simulink model "bike_model_old"  (R2018b)
settings: Solver=VariableStepAuto  StartTime=0.0  StopTime=sim_time  FixedStep=Ts_IMU  MaxStep=Ts  RelTol=1e-3
values from neighbouring files (symbols this model uses):
  a_compFilter = b_compFilter - 0.77    (= 0.325)    [configuration.m]    (also in configuration_pidTuning.m)
  A_kalman = [1 0 Ts 0; 0 1 0 Ts; 0 0 1 0; 0 0 0 1]    [configuration.m]    (also in configuration_pidTuning.m)
  b_compFilter = 1.095    [configuration.m]    (also in configuration_pidTuning.m)
  B_kalman = [0 0 0 0; 0 0 0 0; 0 0 0 0; 0 0 0 0]    [configuration.m]    (also in configuration_pidTuning.m)
  b_real = 1.095    [configuration.m]    (also in configuration_pidTuning.m)
  C_kalman = [1 0 0 0; 0 1 0 0; 0 0 1 0; 0 0 0 1]    [configuration.m]    (also in configuration_pidTuning.m)
  complementary = 0.985    [configuration.m]    (also in configuration_pidTuning.m)
  D_kalman = [0 0 0 0; 0 0 0 0; 0 0 0 0; 0 0 0 0]    [configuration.m]    (also in configuration_pidTuning.m)
  Dead_Band = [0.055, -0.055, 0.005]    [configuration.m]    (also in configuration_pidTuning.m)
  delay = 0.045    [configuration.m]    (also in configuration_pidTuning.m)
  direct_control = 1    [configuration.m]    (also in configuration_pidTuning.m)
  filter_model = 1    [configuration.m]    (also in configuration_pidTuning.m)
  forward_motor_dynamics = 0    [configuration.m]    (also in configuration_pidTuning.m)
  forward_speed_offset = 0    [configuration.m]
  g = 9.81    [configuration.m]    (also in configuration_pidTuning.m)
  I_direct = 0.000227125326188444    (= 0.000227125326188)    [configuration.m]    (also in configuration_pidTuning.m)
  I_lat = 0.000115580509653549    (= 0.000115580509654)    [configuration.m]    (also in configuration_pidTuning.m)
  I_steer = 0.4510120195392    (= 0.451012019539)    [configuration.m]    (also in configuration_pidTuning.m)
  IMU_height_model = 0.45    [configuration.m]    (also in configuration_pidTuning.m)
  IMU_height_real = 0.45    [configuration.m]    (also in configuration_pidTuning.m)
  initial_states = [deg2rad(-2) deg2rad(0) deg2rad(0)]    [configuration.m]    (also in configuration_pidTuning.m)
  input_velocity = 4    [configuration.m]    (also in configuration_pidTuning.m = 3)
  K_dir = [0.2 0 0]    [configuration.m]
  K_pos = [0.02 0 0]    [configuration.m]
  lambda_compFilter = deg2rad(70)    [configuration.m]    (also in configuration_pidTuning.m)
  lambda_real = deg2rad(70)    [configuration.m]    (also in configuration_pidTuning.m)
  lat_control = 0    [configuration.m]    (also in configuration_pidTuning.m = 1)
  look_ahead = 0    [configuration.m]    (also in configuration_pidTuning.m)
  lqr_gains = zeros(length(velocity_lqr),1+size(A_bike,1))    [lqr_design.m]
  max_handlebar = 40*(pi/180)    (= 0.698131700798)    [configuration.m]    (also in configuration_pidTuning.m)
  max_roll = pi/2    (= 1.57079632679)    [configuration.m]    (also in configuration_pidTuning.m)
  max_steering_motor_acc = inf    [configuration.m]    (also in configuration_pidTuning.m)
  max_steering_motor_speed = 0.9    [configuration.m]    (also in configuration_pidTuning.m = 7.5)
  min_handlebar = -max_handlebar    (= -0.698131700798)    [configuration.m]    (also in configuration_pidTuning.m)
  min_roll = - max_roll    (= -1.57079632679)    [configuration.m]    (also in configuration_pidTuning.m)
  min_steering_motor_acc = -inf    [configuration.m]    (also in configuration_pidTuning.m)
  min_steering_motor_speed = -0.9    [configuration.m]    (also in configuration_pidTuning.m = -7.5)
  noise = 0    [configuration.m]    (also in configuration_pidTuning.m)
  noise_acc = 2.4869e-05    [configuration.m]    (also in configuration_pidTuning.m)
  noise_encoder = 1e-7    (= 1e-07)    [configuration.m]    (also in configuration_pidTuning.m)
  noise_gyro = 0.005    [configuration.m]    (also in configuration_pidTuning.m = 0.0022)
  noise_hall = 0.0031    [configuration.m]    (also in configuration_pidTuning.m)
  noise_pos_meas = 0    [configuration.m]    (also in configuration_pidTuning.m = 0.51)
  offset_acc = 0.0*g    (= 0)    [configuration.m]
  offset_encoder = deg2rad(1)    [configuration.m]
  offset_gyro = deg2rad(0)    [configuration.m]
  offset_hall = 0.0    (= 0)    [configuration.m]
  offset_pos_x = 0    [configuration.m]
  offset_pos_y = 0    [configuration.m]
  P_direct = 0.0712859744206787    (= 0.0712859744207)    [configuration.m]    (also in configuration_pidTuning.m)
  P_lat = 0.0465435246389258    (= 0.0465435246389)    [configuration.m]    (also in configuration_pidTuning.m)
  P_steer = 0.219020351848633    (= 0.219020351849)    [configuration.m]    (also in configuration_pidTuning.m)
  parameters_compFilter = [g h_compFilter b_compFilter a_compFilter lambda_compFilter c_compFilter]    [configuration.m]    (also in configuration_pidTuning.m)
  parameters_f_b_real = [m_frame_real m_box_real h_frame_real h_box_real a_frame_real a_box_real c_frame_real c_box_real b_frame_real b_box_real l_frame_real l_box_real]    [configuration.m]    (also in configuration_pidTuning.m)
  parameters_real = [g h_real b_real a_real lambda_real c_real]    [configuration.m]    (also in configuration_pidTuning.m)
  path_tracking = 0    [configuration.m]    (also in configuration_pidTuning.m = 1)
  plant_model = 2    [configuration.m]    (also in configuration_pidTuning.m = 1)
  R_kalman = [noise_pos_meas 0 0 0; 0 noise_pos_meas 0 0; 0 0 noise_hall 0; 0 0 0 noise_hall]    [configuration.m]    (also in configuration_pidTuning.m)
  roll_rate_coef = 0.9    [configuration.m]    (also in configuration_pidTuning.m)
  sensor_offset = 0    [configuration.m]
  steer_control = 0    [configuration.m]    (also in configuration_pidTuning.m = 1)
  steering_angle_correction = deg2rad(0)    [configuration.m]
  steering_motor_limitations = 0    [configuration.m]    (also in configuration_pidTuning.m = 1)
  sys_con = ss(A_lqr,B_lqr,C_lqr,D_lqr)    [lqr_design.m]
  sys_dis = c2d(sys_con,Ts)    [lqr_design.m]
  time_offset_acc = 7    [configuration.m]
  time_offset_encoder = 10    [configuration.m]
  time_offset_gyro = 7    [configuration.m]
  time_offset_hall = 7    [configuration.m]
  time_offset_pos_x = 7    [configuration.m]
  time_offset_pos_y = 7    [configuration.m]
  Ts = 0.01    [configuration.m]    (also in configuration_pidTuning.m = 0.04)
  Ts_IMU = 0.01    [configuration.m]    (also in configuration_pidTuning.m = 0.04)
  uneven_mass = 0    [configuration.m]
  velocity_lqr = [input_velocity - 0.1 , input_velocity , input_velocity + 0.1]    [lqr_design.m]
undefined symbols (not defined in the file or in its folder): A, B, cumulative_dist_along_path, curvature, DiscIntNeverNeededParam, Discrete, initial_x, initial_y, path_x, path_y, Time
libraries: simulink x23, simulink_extras x4, dspsigops x2, ctrlSharedLib x1
(part 3 of 3)

== system bike_model_old/Reference Position /Variable Look Ahead ==
  Velocity : Inport
  Total Tavelled Distance : Inport  Port=2
  1-D Lookup Table2 : Lookup_n-D  NumberOfTableDimensions=1  BreakpointsForDimension1=cumulative_dist_along_path  Table=curvature  ExtrapMethod=Clip  DiagnosticForOutOfRangeInput=Error  InternalRulePriority=Speed  RndMeth=Simplest  InputSameDT=on
  Add1 : Sum
  Clock : Clock
  Delay : Delay  DelayLength=1
  Delay1 : Delay  DelayLength=1
  Demux3 : Demux  Outputs=2
  Gain : Gain  Gain=8
  Look Ahead Time for Curvature Check : Gain  Gain=3
  Look-Ahead Coefficient Selector : MATLAB Function  TreatAsAtomicUnit=on
  "Look-Ahead Coefficient Modifier (Slow Turn-Off) " : MATLAB Function  TreatAsAtomicUnit=on
  Mux1 : Mux  Inputs=2
  Product3 : Product
  Scope2 : Scope
  Look Ahead Distance : Outport
  wires:
  Look Ahead Time for Curvature Check/1 -> Add1/1
  Delay/1 -> "Look-Ahead Coefficient Modifier (Slow Turn-Off) "/2(feedback)
  "Look-Ahead Coefficient Modifier (Slow Turn-Off) "/1(look_ahead_modified) -> Delay/1, Gain/1
  Demux3/1 -> Look-Ahead Coefficient Selector/1(curv_next)
  Look-Ahead Coefficient Selector/1(look_ahead) -> "Look-Ahead Coefficient Modifier (Slow Turn-Off) "/1(look_ahead), Scope2/1
  Clock/1 -> "Look-Ahead Coefficient Modifier (Slow Turn-Off) "/3(time), Delay1/1
  Delay1/1 -> "Look-Ahead Coefficient Modifier (Slow Turn-Off) "/4(time_delayed)
  1-D Lookup Table2/1 -> Demux3/1
  Total Tavelled Distance/1 -> Add1/2, Mux1/2
  Demux3/2 -> Look-Ahead Coefficient Selector/2(curv)
  Gain/1 -> Product3/1  "Look-Ahead Time"
  Add1/1 -> Mux1/1
  Mux1/1 -> 1-D Lookup Table2/1
  Velocity/1 -> Product3/2, Look Ahead Time for Curvature Check/1
  Product3/1 -> Look Ahead Distance/1

== system bike_model_old/Steering Motor/Motor Deadband ==
  Calculated Input : Inport
  Abs : Abs
  Abs1 : Abs
  Constant : Constant  Value=0  SampleTime=Ts
  Constant1 : Constant  Value=0  SampleTime=Ts
  Constant2 : Constant  Value=Dead_Band(2)  SampleTime=Ts
  Constant4 : Constant  Value=Dead_Band(1)  SampleTime=Ts
  Gain : Gain  Gain=-1
  Relay1 : Relay  OnSwitchValue=Dead_Band(3)  OffSwitchValue=-Dead_Band(3)
  Relay2 : Relay  OnSwitchValue=Dead_Band(3)  OffSwitchValue=-Dead_Band(3)
  Sum1 : Sum  Inputs=-+|
  Sum2 : Sum  Inputs=-+|
  Switch : Switch  Criteria=u2 > Threshold
  Switch1 : Switch  Criteria=u2 > Threshold
  Switch2 : Switch  Criteria=u2 > Threshold
  Input Signal After Dead Band : Outport
  wires:
  Constant4/1 -> Sum1/1
  Sum1/1 -> Relay1/1
  Relay1/1 -> Switch/2
  Switch/1 -> Switch1/1
  Constant/1 -> Switch/3
  Switch1/1 -> Input Signal After Dead Band/1
  Switch2/1 -> Switch1/3
  Constant1/1 -> Switch2/3
  Gain/1 -> Sum2/1
  Calculated Input/1 -> Abs/1, Switch2/1, Abs1/1, Switch/1, Switch1/2
  Sum2/1 -> Relay2/1
  Relay2/1 -> Switch2/2
  Abs/1 -> Sum2/2
  Abs1/1 -> Sum1/2
  Constant2/1 -> Gain/1

== system bike_model_old/Steering Motor/Velocity Saturation wrt Max and Min Handle Bar Angles ==
  Reference Steering Rate : Inport
  States : Inport  Port=2
  AND : Logic  IconShape=distinctive  AllPortsSameDT=off  OutDataTypeStr=boolean
  AND1 : Logic  IconShape=distinctive  AllPortsSameDT=off  OutDataTypeStr=boolean
  Compare To Constant : simulink/Logic and Bit Operations/Compare To Constant  relop=>=  const=max_handlebar  OutDataTypeStr=boolean
  Compare To Constant1 : simulink/Logic and Bit Operations/Compare To Constant  relop=<=  const=min_handlebar  OutDataTypeStr=boolean
  Compare To Zero : simulink/Logic and Bit Operations/Compare To Zero  relop=>=  OutDataTypeStr=boolean
  Compare To Zero1 : simulink/Logic and Bit Operations/Compare To Zero  relop=<=  OutDataTypeStr=boolean
  Constant : Constant  Value=0
  Demux : Demux  Outputs=3
  OR : Logic  Operator=OR  IconShape=distinctive  AllPortsSameDT=off  OutDataTypeStr=boolean
  Switch : Switch  Criteria=u2 > Threshold
  Output Steering Rate : Outport
  wires:
  Switch/1 -> Output Steering Rate/1
  Constant/1 -> Switch/1
  States/1 -> Demux/1
  Compare To Constant/1 -> AND/2
  OR/1 -> Switch/2
  Reference Steering Rate/1 -> Switch/3, Compare To Zero/1, Compare To Zero1/1
  Compare To Constant1/1 -> AND1/1
  AND1/1 -> OR/2
  Demux/2 -> Compare To Constant/1, Compare To Constant1/1
  AND/1 -> OR/1
  Compare To Zero1/1 -> AND1/2
  Compare To Zero/1 -> AND/1

== system bike_model_old/Complementary filter/Roll Angle Estimation of Accelerometer/Centripetal Acceleration Compensator ==
  Steering Angle : Inport
  Velocity : Inport  Port=2
  Bike Model b : Constant  Value=b_compFilter
  Divide : Product  Inputs=*/
  Gain : Gain  Gain=sin(lambda_compFilter)
  Multiply : Product
  Square : Math  Operator=square  SaturateOnIntegerOverflow=on
  Tan : Trigonometry  Operator=tan
  Estimated Centripetal Acceleration : Outport
  wires:
  Velocity/1 -> Square/1
  Square/1 -> Divide/1
  Bike Model b/1 -> Divide/2
  Steering Angle/1 -> Gain/1
  Divide/1 -> Multiply/1
  Tan/1 -> Multiply/2
  Multiply/1 -> Estimated Centripetal Acceleration/1
  Gain/1 -> Tan/1

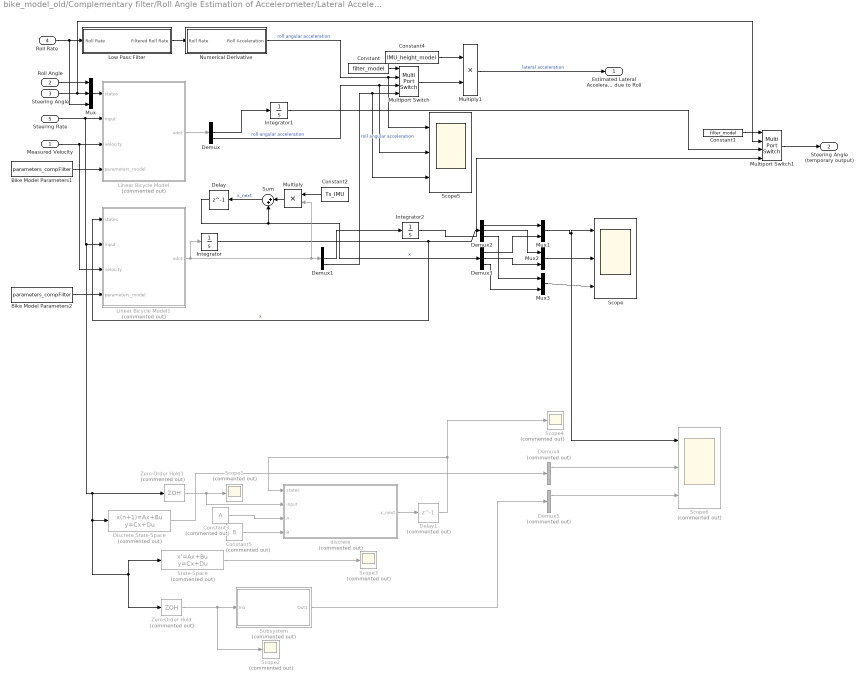
== system bike_model_old/Complementary filter/Roll Angle Estimation of Accelerometer/Lateral Acceleration Compensator ==
  Measured Velocity : Inport
  Roll Angle : Inport  Port=2
  Steering Angle : Inport  Port=3
  Roll Rate : Inport  Port=4
  Steering Rate : Inport  Port=5
  Bike Model Parameters1 : Constant  Value=parameters_compFilter
  Bike Model Parameters2 : Constant  Value=parameters_compFilter
  Constant : Constant  Value=filter_model
  Constant1 : Constant  Value=filter_model
  Constant2 : Constant  Value=Ts_IMU  SampleTime=Ts_IMU
  Constant3 : Constant  Commented=on  Value=A
  Constant4 : Constant  Value=IMU_height_model
  Constant5 : Constant  Commented=on  Value=B
  Delay : Delay  DelayLength=1  InitialCondition=[0 0 0]  SampleTime=Ts_IMU
  Delay1 : Delay  Commented=on  DelayLength=1  InitialCondition=[0 0 0]  SampleTime=Ts_IMU
  Demux{,1..3} (4 alike) : Demux  Outputs=3
  Demux4 : Demux  Commented=on  Outputs=3
  Demux5 : Demux  Commented=on  Outputs=3
  Discrete State-Space : DiscreteStateSpace  Commented=on  A=A  B=B  C=eye(3,3)  D=zeros(3,1)  InitialCondition=[0 0 0]  SampleTime=Ts_IMU
  Integrator : Integrator  InitialCondition=initial_states
  Integrator1 : Integrator  InitialCondition=initial_states(2)
  Integrator2 : Integrator  InitialCondition=initial_states(2)
  Linear Bicycle Model : MATLAB Function  Commented=on  TreatAsAtomicUnit=on
  Linear Bicycle Model1 : MATLAB Function  Commented=on  TreatAsAtomicUnit=on
  Low Pass Filter : Subsystem
  Multiply : Product
  Multiply1 : Product
  Multiport Switch : MultiPortSwitch
  Multiport Switch1 : MultiPortSwitch
  Mux : Mux  Inputs=3
  Mux1 : Mux  Inputs=2
  Mux2 : Mux  Inputs=2
  Mux3 : Mux  Inputs=2
  Numerical Derivative : Subsystem
  Scope : Scope  NumInputPorts=3
  Scope{1..4} (4 alike) : Scope  Commented=on
  Scope5 : Scope  NumInputPorts=3
  Scope6 : Scope  Commented=on  NumInputPorts=3
  State-Space : StateSpace  Commented=on  A=sys_con.A  B=sys_con.B  C=eye(3,3)  D=zeros(3,1)  InitialCondition=[0 0 0]
  Subsystem : Subsystem  Commented=on  TreatAsAtomicUnit=on  SystemSampleTime=Ts_IMU
  Sum : Sum  Inputs=|++
  Zero-Order Hold : ZeroOrderHold  Commented=on  SampleTime=Ts_IMU
  Zero-Order Hold1 : ZeroOrderHold  Commented=on  SampleTime=Ts_IMU
  discrete : MATLAB Function  Commented=on  TreatAsAtomicUnit=on
  Estimated Lateral Accelerattion due to Roll : Outport
  Steering Angle (temporary output) : Outport  Port=2
  wires:
  Numerical Derivative/1(Roll Acceleration) -> Scope5/1, Multiport Switch/2  "roll angular acceleration"
  Roll Rate/1 -> Mux/3, Low Pass Filter/1(Roll Rate)
  Constant4/1 -> Multiply1/1
  Multiply1/1 -> Estimated Lateral Accelerattion due to Roll/1  "lateral acceleration"
  Low Pass Filter/1(Filtered Roll Rate) -> Numerical Derivative/1(Roll Rate)
  Linear Bicycle Model/1(xdot) -> Demux/1
  Demux/3 -> Scope5/2, Multiport Switch/3  "roll angular acceleration"
  Bike Model Parameters1/1 -> Linear Bicycle Model/4(parameters_model)
  Measured Velocity/1 -> Linear Bicycle Model1/3(velocity), Linear Bicycle Model/3(velocity)
  Mux/1 -> Linear Bicycle Model/1(states)
  Roll Angle/1 -> Mux/1
  Steering Angle/1 -> Multiport Switch1/2, Mux/2
  Constant/1 -> Multiport Switch/1
  Multiport Switch/1 -> Multiply1/2
  Demux1/3 -> Scope5/3, Multiport Switch/4  "roll angular acceleration"
  Bike Model Parameters2/1 -> Linear Bicycle Model1/4(parameters_model)
  Delay/1 -> Demux3/1, Sum/2  "x"
  Multiply/1 -> Sum/1
  Constant2/1 -> Multiply/1
  Integrator/1 -> Linear Bicycle Model1/1(states), Demux2/1  "x"
  Demux2/1 -> Mux1/1
  Demux3/1 -> Mux1/2
  Demux2/2 -> Mux2/1
  Demux3/2 -> Mux2/2
  Demux2/3 -> Mux3/1
  Demux3/3 -> Mux3/2
  Mux2/1 -> Scope/2
  Mux1/1 -> Scope6/1, Scope/1
  Mux3/1 -> Scope/3
  Linear Bicycle Model1/1(xdot) -> Multiply/2, Demux1/1, Integrator/1
  State-Space/1 -> Scope3/1
  Delay1/1 -> Scope4/1, discrete/1(states)
  Zero-Order Hold/1 -> Scope2/1, Subsystem/1(In1)
  discrete/1(x_next) -> Delay1/1
  Constant5/1 -> discrete/4(B)
  Constant3/1 -> discrete/3(A)
  Sum/1 -> Delay/1  "x_next"
  Zero-Order Hold1/1 -> discrete/2(input), Scope1/1
  Multiport Switch1/1 -> Steering Angle (temporary output)/1
  Constant1/1 -> Multiport Switch1/1
  Steering Rate/1 -> Zero-Order Hold/1, State-Space/1, Discrete State-Space/1, Zero-Order Hold1/1, Linear Bicycle Model1/2(input), Linear Bicycle Model/2(input)
  Integrator1/1 -> Multiport Switch1/3
  Demux/2 -> Integrator1/1
  Demux1/2 -> Integrator2/1
  Integrator2/1 -> Multiport Switch1/4
  Demux4/1 -> Scope6/2
  Demux5/1 -> Scope6/3
  Discrete State-Space/1 -> Demux4/1
  Subsystem/1(Out1) -> Demux5/1

== system bike_model_old/Path Tracking Controller PID Tuning 2/Tuning of Lateral Position Control/Lateral Error ==
  Psi Sigma : Inport
  Position Error (X,Y) : Inport  Port=2
  Cos : Trigonometry  Operator=cos
  Demux : Demux  Outputs=2
  Product : Product
  Product1 : Product
  Sin : Trigonometry
  Sum : Sum  Inputs=+-|
  To Workspace4 : ToWorkspace  VariableName=LAT_ERR  SaveFormat=Timeseries  SampleTime=Ts
  Lateral Error : Outport
  wires:
  Cos/1 -> Product/2
  Sin/1 -> Product1/1
  Psi Sigma/1 -> Cos/1, Sin/1
  Product1/1 -> Sum/2
  Product/1 -> Sum/1
  Sum/1 -> To Workspace4/1, Lateral Error/1  "Lateral Error"
  Demux/1 -> Product1/2  "X Position Error"
  Demux/2 -> Product/1  "Y Position Error"
  Position Error (X,Y)/1 -> Demux/1

== system bike_model_old/Path Tracking Controller PID Tuning 2/Tuning of Lateral Position Control1/Lateral Error ==
  Psi Sigma : Inport
  Position Error (X,Y) : Inport  Port=2
  Cos : Trigonometry  Operator=cos
  Demux : Demux  Outputs=2
  Product : Product
  Product1 : Product
  Sin : Trigonometry
  Sum : Sum  Inputs=+-|
  Lateral Error : Outport
  wires:
  Cos/1 -> Product/2
  Sin/1 -> Product1/1
  Psi Sigma/1 -> Cos/1, Sin/1
  Product1/1 -> Sum/2
  Product/1 -> Sum/1
  Sum/1 -> Lateral Error/1  "Lateral Error"
  Demux/1 -> Product1/2  "X Position Error"
  Demux/2 -> Product/1  "Y Position Error"
  Position Error (X,Y)/1 -> Demux/1

== system bike_model_old/Physical Bike/Global Angles and Coordinates Calculator - Position/Measured Bike Angles to Global Angles ==
  Velocity : Inport
  Measured Steering Angle : Inport  Port=2
  " Bike Parameters Model " : Constant  Value=parameters_compFilter
  Integrator : Integrator
  MATLAB Function : MATLAB Function  TreatAsAtomicUnit=on
  To Workspace6 : ToWorkspace  VariableName=PSI  SaveFormat=Timeseries  SampleTime=Ts
  To Workspace7 : ToWorkspace  VariableName=BETA  SaveFormat=Timeseries  SampleTime=Ts
  Psi : Outport
  Beta : Outport  Port=2
  wires:
  MATLAB Function/2(beta) -> Beta/1, To Workspace7/1
  MATLAB Function/1(psi_d) -> Integrator/1
  Integrator/1 -> Psi/1, To Workspace6/1
  " Bike Parameters Model "/1 -> MATLAB Function/2(parameters_model)
  Measured Steering Angle/1 -> MATLAB Function/3(delta)
  Velocity/1 -> MATLAB Function/1(v)

== system bike_model_old/Physical Bike/Global Angles and Coordinates Calculator - Position/Measured Global Angles to Global Coordinates ==
  Velocity : Inport
  Psi : Inport  Port=2
  Beta : Inport  Port=3
  Constant : Constant  Value=initial_y
  Constant1 : Constant  Value=initial_x
  Integrator1 : Integrator
  Integrator2 : Integrator
  MATLAB Function1 : MATLAB Function  TreatAsAtomicUnit=on
  Mux : Mux  Inputs=2
  Sum : Sum  Inputs=|++
  Sum1 : Sum  Inputs=++|
  "Position (X, Y)" : Outport
  wires:
  MATLAB Function1/2(Ydot) -> Integrator2/1  "Ydot"
  MATLAB Function1/1(Xdot) -> Integrator1/1  "Xdot"
  Psi/1 -> MATLAB Function1/2(psi)
  Beta/1 -> MATLAB Function1/3(beta)
  Velocity/1 -> MATLAB Function1/1(v)
  Integrator2/1 -> Sum/1
  Constant/1 -> Sum/2
  Sum/1 -> Mux/2
  Integrator1/1 -> Sum1/2
  Sum1/1 -> Mux/1
  Constant1/1 -> Sum1/1
  Mux/1 -> "Position (X, Y)"/1

== system bike_model_old/Complementary filter/Roll Angle Estimation of Accelerometer/Lateral Acceleration Compensator/Low Pass Filter ==
  Roll Rate : Inport
  Delay18 : Delay  DelayLength=1
  Gain4 : Gain  Gain=roll_rate_coef
  Gain6 : Gain  Gain=1-roll_rate_coef
  Scope7 : Scope  NumInputPorts=2
  Sum4 : Sum  Inputs=|++
  Filtered Roll Rate : Outport
  wires:
  Gain6/1 -> Sum4/1
  Gain4/1 -> Sum4/2
  Sum4/1 -> Filtered Roll Rate/1, Delay18/1, Scope7/2  "Filtered Roll Rate"
  Delay18/1 -> Gain4/1
  Roll Rate/1 -> Scope7/1, Gain6/1  "Measured Roll Rate"

== system bike_model_old/Complementary filter/Roll Angle Estimation of Accelerometer/Lateral Acceleration Compensator/Numerical Derivative ==
  Roll Rate : Inport
  Delay18 : Delay  DelayLength=1
  Gain3 : Gain  Gain=1/Ts_IMU
  Sum3 : Sum  Inputs=|+-
  Roll Acceleration : Outport
  wires:
  Sum3/1 -> Gain3/1
  Delay18/1 -> Sum3/2
  Roll Rate/1 -> Sum3/1, Delay18/1
  Gain3/1 -> Roll Acceleration/1

== system bike_model_old/Complementary filter/Roll Angle Estimation of Accelerometer/Lateral Acceleration Compensator/Subsystem ==
  In1 : Inport
  Constant : Constant  Value=A
  Constant1 : Constant  Value=B
  Delay1 : Delay  DelayLength=1  InitialCondition=[0 0 0]  SampleTime=Ts_IMU
  Multiply : Product  Multiplication=Matrix(*)
  Multiply1 : Product  Multiplication=Matrix(*)
  Sum2 : Sum  Inputs=|++
  Out1 : Outport
  wires:
  Sum2/1 -> Delay1/1
  Multiply1/1 -> Sum2/2
  In1/1 -> Multiply1/2  "u"
  Delay1/1 -> Multiply/2, Out1/1  "x"
  Multiply/1 -> Sum2/1
  Constant/1 -> Multiply/1
  Constant1/1 -> Multiply1/1

== matlab function bike_model_old/Balance Controller/Reference States/Reference Roll Angle Calculator ==
  data: parameters_real input; velocity input; delta_ref input; phi_ref output
function phi_ref = fcn(parameters_real, velocity, delta_ref)
g = parameters_real(1);
b = parameters_real(3);
v = velocity;

phi_ref = -atan(v^2 / (g * b) * delta_ref); % tan(theta_ref));

== matlab function bike_model_old/Physical Bike/Linear Bicycle Model ==
  data: states input; input input; xdot output; velocity input; disturbance input; parameters_real input; parameters_f_b_real input
function xdot = fcn(states,input,velocity,disturbance,parameters_real,parameters_f_b_real)

delta_d=input;
v=velocity;
d1=disturbance(1);
d2=disturbance(2);
d3=disturbance(3);

% 1=frame | 2=box
m1=parameters_f_b_real(1);
m2=parameters_f_b_real(2);
h1=parameters_f_b_real(3);
h2=parameters_f_b_real(4);
a1=parameters_f_b_real(5);
a2=parameters_f_b_real(6);
c1=parameters_f_b_real(7);
c2=parameters_f_b_real(8);
b1=parameters_f_b_real(9);
b2=parameters_f_b_real(10);
l1=parameters_f_b_real(11);
l2=parameters_f_b_real(12);

g=parameters_real(1);
%h=parameters_real(2);
b=parameters_real(3);
%a=parameters_real(4);
lambda=parameters_real(5);
c=parameters_real(6);

phi=states(1);
delta=states(2);
phi_d=states(3);

A=((m1/12)*((c1^2)+(b1^2)))+(m1*(h1^2))+((m2/12)*((c2^2)+(b2^2)))+(m2*(h2^2));
B=((m1/12)*((l1^2)+(b1^2)))-(m1*a1*h1)+((m2/12)*((c2^2)+(b2^2)))+(m2*a2*h2);
D=(((m1*h1)+(m2*h2))*(v^2))-(c*g*((m1*a1)-(m2*a2)));

xdot1=phi_d+d1;
xdot2=delta_d+d2;
xdot3=((((m1*h1)+(m2*h2))*g)/A)*phi+((D*sin(lambda))/(b*A))*delta+d3+((B*v*sin(lambda))/(b*A))*delta_d;

xdot=[xdot1 xdot2 xdot3];

== matlab function bike_model_old/Global Angles and Coordinates Calculator - Position/Measured Bike Angles to Global Angles/MATLAB Function ==
  data: v input; parameters_model input; delta input; psi_d output; beta output
function [psi_d, beta]  = fcn(v, parameters_model, delta)

b = parameters_model(3);
a = parameters_model(4);

beta = atan((a / (b)) * tan(delta));
psi_d = (v / a) * sin(beta);

== matlab function bike_model_old/Reference Position /Variable Look Ahead/Look-Ahead Coefficient Modifier (Slow Turn-Off)  ==
  data: look_ahead input; look_ahead_modified output; feedback input; time input; time_delayed input
function look_ahead_modified = fcn(look_ahead, feedback, time, time_delayed)

step=time-time_delayed;

kill_time=3;

delta=(feedback*step)/kill_time;

if look_ahead-feedback<-0.0001
    look_ahead_modified=feedback-delta;
else
    look_ahead_modified = look_ahead;
end
    

end

== matlab function bike_model_old/Global Angles and Coordinates Calculator - Position/Measured Global Angles to Global Coordinates/MATLAB Function1 ==
  data: v input; psi input; Xdot output; beta input; Ydot output
function [Xdot, Ydot]  = fcn(v, psi, beta)

Xdot = v * cos(psi + beta);
Ydot = v * sin(psi + beta);

== matlab function bike_model_old/Reference Position /Variable Look Ahead/Look-Ahead Coefficient Selector ==
  data: curv_next input; look_ahead output; curv input
function look_ahead = fcn(curv_next, curv)


if curv>-0.01 && curv<0.01
    curv=0;
end

if curv_next>-0.01 && curv_next<0.01
    curv_next=0;
end



if curv>=0
    if curv-curv_next>0
        look_ahead=0;
    else
        look_ahead=curv_next-curv;
    end
else
    if curv-curv_next<0
        look_ahead=0;
    else
        look_ahead=curv-curv_next;
    end
end



end

== matlab function bike_model_old/Complementary filter/Roll Angle Estimation of Accelerometer/Lateral Acceleration Compensator/Linear Bicycle Model ==
  data: states input; input input; xdot output; velocity input; parameters_model input
function xdot = fcn(states,input,velocity,parameters_model)

delta_d=input;
v=velocity;

g=parameters_model(1);
h=parameters_model(2);
b=parameters_model(3);
a=parameters_model(4);
lambda=parameters_model(5);
c=parameters_model(6);

phi=states(1);
delta=states(2);
phi_d=states(3);

xdot1=phi_d;
xdot2=delta_d;
xdot3=(g/h)*phi+((a*v)/(b*h))*sin(lambda)*delta_d+((h*v^2-g*a*c)/(b*h^2))*sin(lambda)*delta;

xdot=[xdot1 xdot2 xdot3];

== matlab function bike_model_old/Physical Bike/Global Angles and Coordinates Calculator - Position/Measured Bike Angles to Global Angles/MATLAB Function ==
  data: v input; parameters_model input; delta input; psi_d output; beta output
function [psi_d, beta]  = fcn(v, parameters_model, delta)

b = parameters_model(3);
a = parameters_model(4);

beta = atan((a / (b)) * tan(delta));
psi_d = (v / a) * sin(beta);

== matlab function bike_model_old/Physical Bike/Nonlinear Bicycle Model ==
  data: states input; input input; xdot output; velocity input; disturbance input; parameters_real input; parameters_f_b_real input; uneven_mass input
function xdot = fcn(states,input,velocity,disturbance,parameters_real,parameters_f_b_real,uneven_mass)

delta_d=input;
v=velocity;
d1=disturbance(1);
d2=disturbance(2);
d3=disturbance(3);

% 1=frame | 2=box
m1=parameters_f_b_real(1);
m2=parameters_f_b_real(2);
h1=parameters_f_b_real(3);
h2=parameters_f_b_real(4);
a1=parameters_f_b_real(5);
a2=parameters_f_b_real(6);
c1=parameters_f_b_real(7);
c2=parameters_f_b_real(8);
b1=parameters_f_b_real(9);
b2=parameters_f_b_real(10);
l1=parameters_f_b_real(11);
l2=parameters_f_b_real(12);

g=parameters_real(1);
%h=parameters_real(2);
b=parameters_real(3);
%a=parameters_real(4);
lambda=parameters_real(5);
c=parameters_real(6);

A=((m1/12)*((c1^2)+(b1^2)))+(m1*(h1^2))+((m2/12)*((c2^2)+(b2^2)))+(m2*(h2^2));
B=(m1*a1*h1)-(m2*a2*h2);
D=(((m1*h1)+(m2*h2))*(v^2))-(c*g*((m1*a1)-(m2*a2)));

phi=states(1);
delta=states(2);
phi_d=states(3);

% Biaised mass from box mass measurement
% if uneven_mass
%     m = 9.3;
%     d = 0.03;
%     T = m*d*g*cos(phi)/A;
% else
%     T = 0;
% end

% Biaised mass from bike equilibrium measurement
if uneven_mass
    m = 9.3;
    d = 0.07;
    T = m*d*g*cos(phi)/A;
else
    T = 0;
end

xdot1=phi_d+d1;
xdot2=delta_d+d2;
xdot3=((((m1*h1)+(m2*h2))*g)/A)*tan(phi) - T +((D*sin(lambda))/(b*A))*tan(delta)+d3+((B*v*sin(lambda))/(b*A))*tan(delta_d);

xdot=[xdot1 xdot2 xdot3];

== matlab function bike_model_old/Physical Bike/Linear Bicycle Model with neglected fork angle (lambda=90deg, c=0) "THE SIMPLEST MODEL" ==
  data: states input; input input; xdot output; velocity input; disturbance input; parameters_real input; parameters_f_b_real input
function xdot = fcn(states,input,velocity,disturbance,parameters_real,parameters_f_b_real)

delta_d=input;
v=velocity;
d1=disturbance(1);
d2=disturbance(2);
d3=disturbance(3);

% 1=frame | 2=box
m1=parameters_f_b_real(1);
m2=parameters_f_b_real(2);
h1=parameters_f_b_real(3);
h2=parameters_f_b_real(4);
a1=parameters_f_b_real(5);
a2=parameters_f_b_real(6);
c1=parameters_f_b_real(7);
c2=parameters_f_b_real(8);
b1=parameters_f_b_real(9);
b2=parameters_f_b_real(10);
l1=parameters_f_b_real(11);
l2=parameters_f_b_real(12);

g=parameters_real(1);
%h=parameters_real(2);
b=parameters_real(3);
%a=parameters_real(4);
lambda=parameters_real(5);
c=parameters_real(6);

A=((m1/12)*((c1^2)+(b1^2)))+(m1*(h1^2))+((m2/12)*((c2^2)+(b2^2)))+(m2*(h2^2));
B=((m1/12)*((l1^2)+(b1^2)))-(m1*a1*h1)+((m2/12)*((c2^2)+(b2^2)))+(m2*a2*h2);
D=(((m1*h1)+(m2*h2))*(v^2))-(c*g*((m1*a1)-(m2*a2)));

phi=states(1);
delta=states(2);
phi_d=states(3);

xdot1=phi_d+d1;
xdot2=delta_d+d2;
xdot3=((((m1*h1)+(m2*h2))*g)/A)*phi+((D*sin(lambda))/(b*A))*delta+d3+((B*v*sin(lambda))/(b*A))*delta_d;

xdot=[xdot1 xdot2 xdot3];

== matlab function bike_model_old/Global Angles and Coordinates Calculator - Velocity/Measured Bike Angles to Global Angles/MATLAB Function ==
  data: v input; parameters_model input; delta input; psi_d output; beta output
function [psi_d, beta]  = fcn(v, parameters_model, delta)

b = parameters_model(3);
a = parameters_model(4);

beta = atan((a / (b)) * tan(delta));
psi_d = (v / a) * sin(beta);

== matlab function bike_model_old/Complementary filter/Roll Angle Estimation of Accelerometer/Lateral Acceleration Compensator/Linear Bicycle Model1 ==
  data: states input; input input; xdot output; velocity input; parameters_model input
function xdot = fcn(states,input,velocity,parameters_model)

delta_d=input;
v=velocity;

g=parameters_model(1);
h=parameters_model(2);
b=parameters_model(3);
a=parameters_model(4);
lambda=parameters_model(5);
c=parameters_model(6);

phi=states(1);
delta=states(2);
phi_d=states(3);

xdot1=phi_d;
xdot2=delta_d;
xdot3=(g/h)*phi+((a*v)/(b*h))*sin(lambda)*delta_d+((h*v^2-g*a*c)/(b*h^2))*sin(lambda)*delta;

xdot=[xdot1; xdot2; xdot3];

== matlab function bike_model_old/Complementary filter/Roll Angle Estimation of Accelerometer/Lateral Acceleration Compensator/discrete ==
  data: states input; input input; x_next output; A input; B input
function x_next = fcn(states,input,A,B)





x_next=A*states+B*input;

== matlab function bike_model_old/Global Angles and Coordinates Calculator - Velocity/Measured Global Angles to Global Coordinates/MATLAB Function1 ==
  data: v input; psi input; Xdot output; beta input; Ydot output
function [Xdot, Ydot]  = fcn(v, psi, beta)

Xdot = v * cos(psi + beta);
Ydot = v * sin(psi + beta);

== matlab function bike_model_old/Physical Bike/Global Angles and Coordinates Calculator - Position/Measured Global Angles to Global Coordinates/MATLAB Function1 ==
  data: v input; psi input; Xdot output; beta input; Ydot output
function [Xdot, Ydot]  = fcn(v, psi, beta)

Xdot = v * cos(psi + beta);
Ydot = v * sin(psi + beta);
